simulink model "Crazyflie_NoLinealModel_EB"  (R2020b)
settings: Solver=FixedStepAuto  StartTime=0.0  StopTime=30  FixedStep=0.001  RelTol=1e-3
values from neighbouring files (symbols this model uses):
  fm = 0.2685    [Crazyflie_Model.m]
  we = sqrt((m*g)/(4*CT))    [Crazyflie_Model.m]
undefined symbols (not defined in the file or in its folder): DiscIntNeverNeededParam, Dphi_s, Dphi_T, Dpsi_s, Dtheta_s, KIz, magnitude, MCO, Phi_s, Phi_T, phi_theta_limit, quad, Theta_s, U_s, V_s, X_s, X_T, XY_delta, xyv_lim, Y_s, Yaw_delta, Yaw_s, Yaw_T, Z_delta, Z_s, Z_T
libraries: simulink x16, pid_lib x11
(part 1 of 2)
settings Model: Creator=Rafael  LastModifiedBy=FranciscoJose
settings DataIOCC: LimitDataPoints=on  SaveFormat=Array  SignalLoggingSaveFormat=ModelDataLogs  ReturnWorkspaceOutputs=off
settings OptimizationCC: ExpressionDepthLimit=2147483647  LifeSpan=inf
settings DebuggingCC: UnderspecifiedInitializationDetection=Classic  MergeDetectMultiDrivingBlocksExec=none  SolverPrmCheckMsg=warning  FcnCallInpInsideContextMsg=warning  AllowSymbolicDim=off  StateNameClashWarn=warning  SFUnexpectedBacktrackingDiag=warning  SFNoUnconditionalDefaultTransitionDiag=warning  SFExecutionAtInitializationDiag=none  ArithmeticOperatorsInVariantConditions=warning
settings HardwareCC: ProdBitPerPointer=32  ProdBitPerSizeT=32  ProdBitPerPtrDiffT=32  ProdLargestAtomicFloat=None  ProdIntDivRoundTo=Undefined  ProdEndianess=Unspecified  ProdWordSize=32  ProdHWDeviceType=32-bit Generic
settings ModelReferenceCC: PropagateSignalLabelsOutOfModel=off
settings SFSimCC: SimUseLocalCustomCode=off  CustomCodeUndefinedFunction=UseInterfaceOnly
settings RTWCC: RTWUseLocalCustomCode=off
settings CodeAppCC: StateflowObjectComments=on
settings GRTTargetCC: TargetLangStandard=C89/C90 (ANSI)
settings ConfigComp: CovMetricSettings=dw  CovSaveCumulativeToWorkspaceVar=on  CovSaveSingleToWorkspaceVar=on  CovExternalEMLEnable=off
settings SimscapeCC: SimscapeNormalizeSystem=off
settings ConfigurationSet: Description=SimMechanics 2G

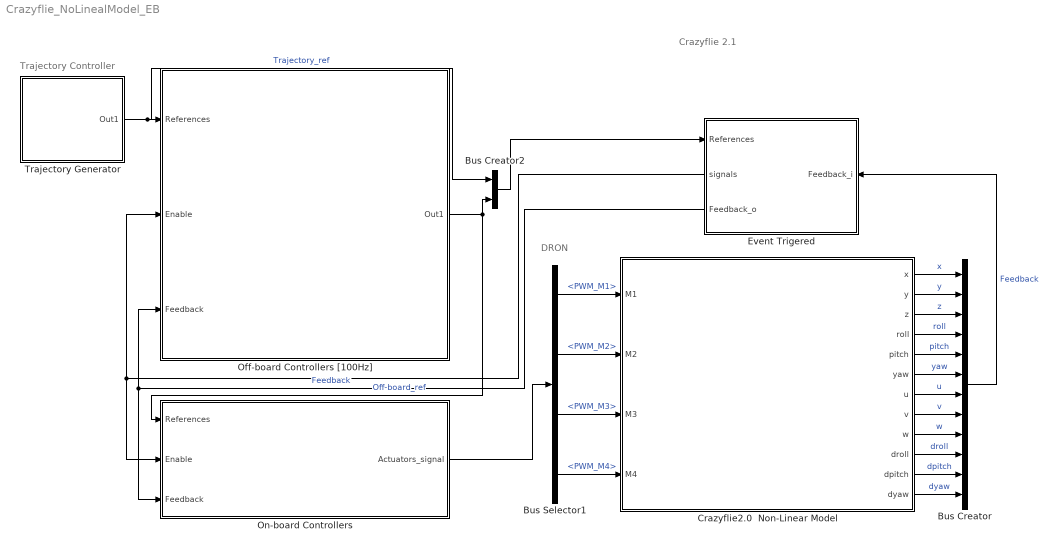
== system Crazyflie_NoLinealModel_EB ==
  note: DRON
  note: Trajectory Controller
  note: Crazyflie 2.1
  Bus Creator : BusCreator  Inputs=12
  Bus Creator2 : BusCreator  Inputs=2
  Bus Selector1 : BusSelector  OutputSignals=PWM_M1,PWM_M2,PWM_M3,PWM_M4
  Crazyflie2.0  Non-Linear Model : Subsystem
      mask Display: image('$imagefile'); % Use "Edit Image" on toolstrip to change.
  Event Trigered : Subsystem
      settings: PortSchema="{\"entries\":[{\"content\":{\"sides\":[{\"content\":{\"connectorIds\":[\"In1\",\"Out1\",\"Out2\"]},\"type\":\"ConnectorPlacement.EquallySpacedRectSide\",\"uuid\":\"5ef058f8-e335-44ad-8d03-d23aa6bafaea\"},{\"content\":{\"connectorIds\":[\"In2\"],\"side\":\"RIGHT\"},\"type\":\"ConnectorPlacement.EquallySpacedRectSide\",\"uuid\":\"829d21a1-bc41-4ced-ab22-24584c4435de\"},{\"content\":{\"connectorIds\":[],\"side\":\"TOP\"},\"type\":\"ConnectorPlacement.EquallySpacedRectSide\",\"uuid\":\"72379b45-c383-4ef8-bce9-8d80bc7025bf\"},{\"content\":{\"connectorIds\":[],\"side\":\"HIDDEN\"},\"type\":\"ConnectorPlacement.EquallySpacedRectSide\",\"uuid\":\"f776fbe7-ec28-4c8f-acaa-997e45e4d7f5\"}]},\"type\":\"ConnectorPlacement.EquallySpacedConnector\",\"uuid\":\"d6c0820c-12f4-49d2-aae7-90f0c967141d\"}],\"packageUris\":[\"http://schema.mathworks.com/mf0/Connector/R2020b\"],\"version\":\"1.0\"}"
  Off-board Controllers [100Hz] : Subsystem
  On-board Controllers : Subsystem
  Trajectory Generator : Subsystem
  wires:
  Crazyflie2.0  Non-Linear Model/11(dpitch) -> Bus Creator/11  "dpitch"
  Crazyflie2.0  Non-Linear Model/3(z) -> Bus Creator/3  "z"
  Crazyflie2.0  Non-Linear Model/12(dyaw) -> Bus Creator/12  "dyaw"
  Crazyflie2.0  Non-Linear Model/4(roll) -> Bus Creator/4  "roll"
  Crazyflie2.0  Non-Linear Model/5(pitch) -> Bus Creator/5  "pitch"
  Crazyflie2.0  Non-Linear Model/6(yaw) -> Bus Creator/6  "yaw"
  Crazyflie2.0  Non-Linear Model/1(x) -> Bus Creator/1  "x"
  Crazyflie2.0  Non-Linear Model/2(y) -> Bus Creator/2  "y"
  Crazyflie2.0  Non-Linear Model/7(u) -> Bus Creator/7  "u"
  Crazyflie2.0  Non-Linear Model/8(v) -> Bus Creator/8  "v"
  Crazyflie2.0  Non-Linear Model/9(w) -> Bus Creator/9  "w"
  Crazyflie2.0  Non-Linear Model/10(droll) -> Bus Creator/10  "droll"
  Event Trigered/2(Feedback_o) -> Off-board Controllers [100Hz]/3(Feedback), On-board Controllers/3(Feedback)  "Feedback"
  Bus Selector1/1 -> Crazyflie2.0  Non-Linear Model/1(M1)  "<PWM_M1>"
  Bus Selector1/2 -> Crazyflie2.0  Non-Linear Model/2(M2)  "<PWM_M2>"
  Bus Selector1/3 -> Crazyflie2.0  Non-Linear Model/3(M3)  "<PWM_M3>"
  Bus Selector1/4 -> Crazyflie2.0  Non-Linear Model/4(M4)  "<PWM_M4>"
  Trajectory Generator/1(Out1) -> Bus Creator2/1, Off-board Controllers [100Hz]/1(References)  "Trajectory_ref"
  Bus Creator2/1 -> Event Trigered/1(References)
  Bus Creator/1 -> Event Trigered/2(Feedback_i)  "Feedback"
  Event Trigered/1(signals) -> On-board Controllers/2(Enable), Off-board Controllers [100Hz]/2(Enable)
  On-board Controllers/1(Actuators_signal) -> Bus Selector1/1
  Off-board Controllers [100Hz]/1(Out1) -> On-board Controllers/1(References), Bus Creator2/2  "Off-board_ref"

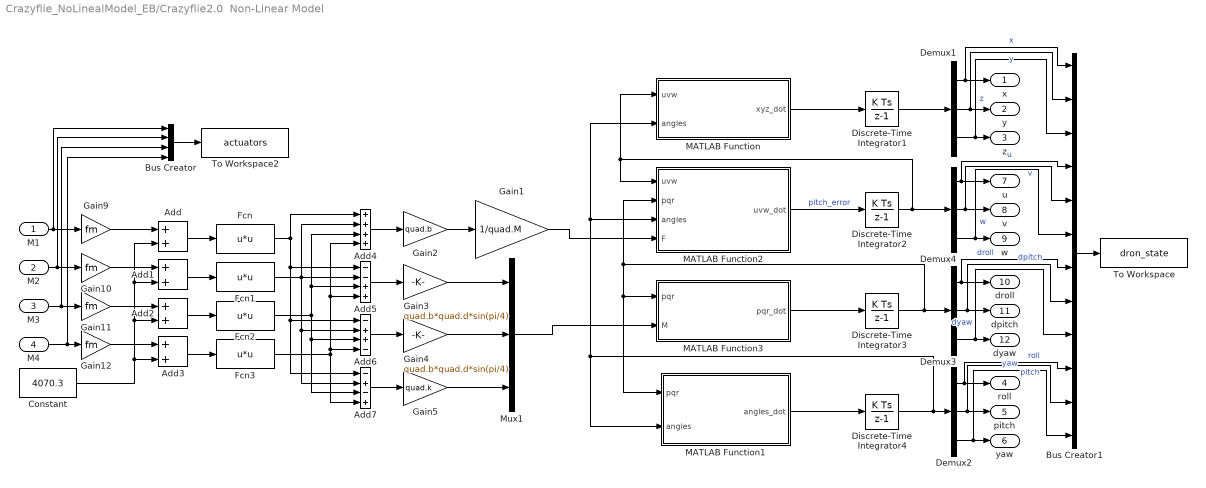
== system Crazyflie_NoLinealModel_EB/Crazyflie2.0  Non-Linear Model ==
  M1 : Inport
  M2 : Inport  Port=2
  M3 : Inport  Port=3
  M4 : Inport  Port=4
  Add{,1..3} (4 alike) : Sum
  Add4 : Sum  Inputs=++++
  Add5 : Sum  Inputs=--++
  Add6 : Sum  Inputs=-++-
  Add7 : Sum  Inputs=-+-+
  Bus Creator : BusCreator  Inputs=4
  Bus Creator1 : BusCreator  Inputs=12
  Constant : Constant  Value=4070.3
  Demux{1..4} (4 alike) : Demux  Outputs=3
  Discrete-Time Integrator{1..4} (4 alike) : DiscreteIntegrator  SampleTime=0.001  ICPrevOutput=DiscIntNeverNeededParam  ICPrevScaledInput=DiscIntNeverNeededParam
  Fcn{,1..3} (4 alike) : Fcn  Expr=u*u
  Gain1 : Gain  Gain=1/quad.M
  Gain{9..12} (4 alike) : Gain  Gain=fm
  Gain2 : Gain  Gain=quad.b
  Gain3 : Gain  Gain=quad.b*quad.d*sin(pi/4)
  Gain4 : Gain  Gain=quad.b*quad.d*sin(pi/4)
  Gain5 : Gain  Gain=quad.k
  MATLAB Function : MATLAB Function  TreatAsAtomicUnit=on
  MATLAB Function1 : MATLAB Function  TreatAsAtomicUnit=on
  MATLAB Function2 : MATLAB Function  TreatAsAtomicUnit=on
  MATLAB Function3 : MATLAB Function  TreatAsAtomicUnit=on
  Mux1 : Mux  Inputs=3
  To Workspace : ToWorkspace  VariableName=dron_state  SaveFormat=Timeseries  SampleTime=-1
  To Workspace2 : ToWorkspace  VariableName=actuators  SaveFormat=Timeseries  SampleTime=-1
  x : Outport
  y : Outport  Port=2
  z : Outport  Port=3
  roll : Outport  Port=4
  pitch : Outport  Port=5
  yaw : Outport  Port=6
  u : Outport  Port=7
  v : Outport  Port=8
  w : Outport  Port=9
  droll : Outport  Port=10
  dpitch : Outport  Port=11
  dyaw : Outport  Port=12
  wires:
  Demux1/1 -> Bus Creator1/1, x/1  "x"
  Demux1/2 -> Bus Creator1/2, y/1  "y"
  Demux1/3 -> Bus Creator1/3, z/1  "z"
  Demux2/1 -> Bus Creator1/10, roll/1  "roll"
  Demux2/2 -> Bus Creator1/11, pitch/1  "pitch"
  Demux2/3 -> Bus Creator1/12, yaw/1  "yaw"
  Demux4/1 -> Bus Creator1/4, u/1  "u"
  Demux4/2 -> Bus Creator1/5, v/1  "v"
  Demux4/3 -> Bus Creator1/6, w/1  "w"
  Demux3/1 -> Bus Creator1/7, droll/1  "droll"
  Demux3/2 -> Bus Creator1/8, dpitch/1  "dpitch"
  Demux3/3 -> Bus Creator1/9, dyaw/1  "dyaw"
  M1/1 -> Bus Creator/1, Gain9/1
  M2/1 -> Gain10/1, Bus Creator/2
  M3/1 -> Bus Creator/3, Gain11/1
  M4/1 -> Bus Creator/4, Gain12/1
  Add/1 -> Fcn/1
  Add1/1 -> Fcn1/1
  Add2/1 -> Fcn2/1
  Add3/1 -> Fcn3/1
  Gain9/1 -> Add/1
  Gain10/1 -> Add1/1
  Gain11/1 -> Add2/1
  Gain12/1 -> Add3/1
  Constant/1 -> Add3/2, Add/2, Add1/2, Add2/2
  Discrete-Time Integrator3/1 -> Demux3/1, MATLAB Function2/2(pqr), MATLAB Function1/1(pqr), MATLAB Function3/1(pqr)
  Discrete-Time Integrator2/1 -> MATLAB Function2/1(uvw), MATLAB Function/1(uvw), Demux4/1
  MATLAB Function3/1(pqr_dot) -> Discrete-Time Integrator3/1
  MATLAB Function1/1(angles_dot) -> Discrete-Time Integrator4/1
  Mux1/1 -> MATLAB Function3/2(M)
  Discrete-Time Integrator4/1 -> Demux2/1, MATLAB Function1/2(angles), MATLAB Function/2(angles), MATLAB Function2/3(angles)
  Discrete-Time Integrator1/1 -> Demux1/1
  MATLAB Function/1(xyz_dot) -> Discrete-Time Integrator1/1
  Gain4/1 -> Mux1/2
  Add6/1 -> Gain4/1
  Gain5/1 -> Mux1/3
  Gain3/1 -> Mux1/1
  Gain1/1 -> MATLAB Function2/4(F)
  Fcn2/1 -> Add4/3, Add5/3, Add7/3, Add6/3
  Add7/1 -> Gain5/1
  Fcn/1 -> Add4/1, Add7/1, Add6/1, Add5/1
  Add5/1 -> Gain3/1
  Fcn3/1 -> Add4/4, Add5/4, Add6/4, Add7/4
  Fcn1/1 -> Add4/2, Add7/2, Add6/2, Add5/2
  Gain2/1 -> Gain1/1
  Add4/1 -> Gain2/1
  MATLAB Function2/1(uvw_dot) -> Discrete-Time Integrator2/1  "pitch_error"
  Bus Creator/1 -> To Workspace2/1
  Bus Creator1/1 -> To Workspace/1

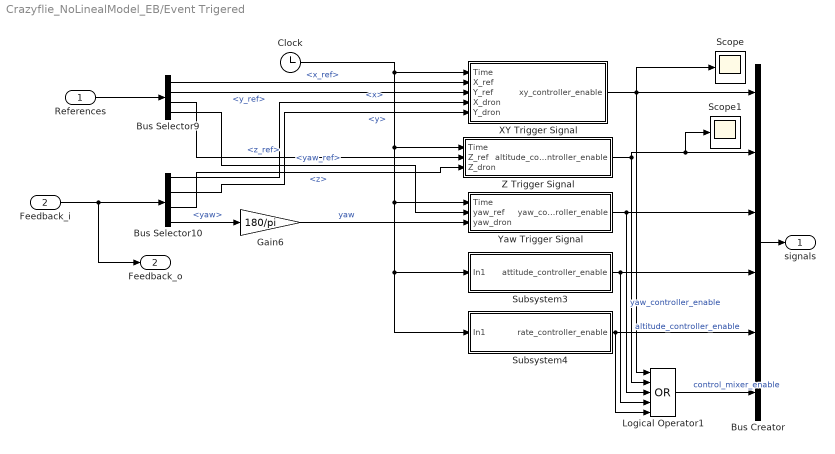
== system Crazyflie_NoLinealModel_EB/Event Trigered ==
  References : Inport
  Feedback_i : Inport  Port=2
  Bus Creator : BusCreator  Inputs=6
  Bus Selector10 : BusSelector  OutputSignals=x,y,z,yaw
  Bus Selector9 : BusSelector  OutputSignals=Trajectory_ref.x_ref,Trajectory_ref.y_ref,Trajectory_ref.z_ref,Trajectory_ref.yaw_ref
  Clock : Clock
  Gain6 : Gain  Gain=180/pi
  Logical Operator1 : Logic  Operator=OR  Inputs=5  AllPortsSameDT=off  OutDataTypeStr=boolean
  Scope : Scope
  Scope1 : Scope
  Subsystem3 : Subsystem
  Subsystem4 : Subsystem
  XY Trigger Signal : Subsystem
  Yaw Trigger Signal : Subsystem
  Z Trigger Signal : Subsystem
  signals : Outport
  Feedback_o : Outport  Port=2
  wires:
  References/1 -> Bus Selector9/1
  Feedback_i/1 -> Bus Selector10/1, Feedback_o/1
  Bus Selector9/1 -> XY Trigger Signal/2(X_ref)  "<x_ref>"
  Bus Selector9/2 -> XY Trigger Signal/3(Y_ref)  "<y_ref>"
  Bus Selector9/4 -> Yaw Trigger Signal/2(yaw_ref)  "<yaw_ref>"
  Bus Selector10/1 -> XY Trigger Signal/4(X_dron)  "<x>"
  Bus Selector10/2 -> XY Trigger Signal/5(Y_dron)  "<y>"
  Bus Selector10/3 -> Z Trigger Signal/3(Z_dron)  "<z>"
  Bus Selector10/4 -> Gain6/1  "<yaw>"
  Bus Selector9/3 -> Z Trigger Signal/2(Z_ref)  "<z_ref>"
  Bus Creator/1 -> signals/1
  Gain6/1 -> Yaw Trigger Signal/3(yaw_dron)  "yaw"
  Logical Operator1/1 -> Bus Creator/6  "control_mixer_enable"
  Z Trigger Signal/1(altitude_controller_enable) -> Scope1/1, Bus Creator/2, Logical Operator1/2  "altitude_controller_enable"
  XY Trigger Signal/1(xy_controller_enable) -> Scope/1, Logical Operator1/1, Bus Creator/1
  Yaw Trigger Signal/1(yaw_controller_enable) -> Logical Operator1/3, Bus Creator/3  "yaw_controller_enable"
  Subsystem3/1(attitude_controller_enable) -> Logical Operator1/4, Bus Creator/4
  Clock/1 -> Subsystem4/1(In1), Subsystem3/1(In1), Yaw Trigger Signal/1(Time), Z Trigger Signal/1(Time), XY Trigger Signal/1(Time)
  Subsystem4/1(rate_controller_enable) -> Logical Operator1/5, Bus Creator/5

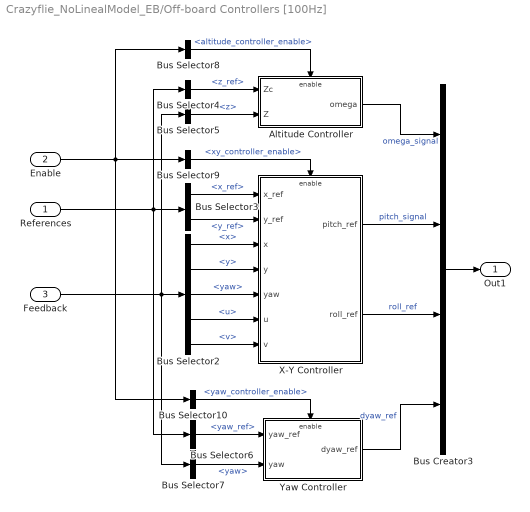
== system Crazyflie_NoLinealModel_EB/Off-board Controllers [100Hz] ==
  References : Inport
  Enable : Inport  Port=2
  Feedback : Inport  Port=3
  Altitude Controller : Subsystem  TreatAsAtomicUnit=on
  Bus Creator3 : BusCreator  Inputs=4
  Bus Selector10 : BusSelector  OutputSignals=yaw_controller_enable
  Bus Selector2 : BusSelector  OutputSignals=x,y,yaw,u,v
  Bus Selector3 : BusSelector  OutputSignals=x_ref,y_ref
  Bus Selector4 : BusSelector  OutputSignals=z_ref
  Bus Selector5 : BusSelector  OutputSignals=z
  Bus Selector6 : BusSelector  OutputSignals=yaw_ref
  Bus Selector7 : BusSelector  OutputSignals=yaw
  Bus Selector8 : BusSelector  OutputSignals=altitude_controller_enable
  Bus Selector9 : BusSelector  OutputSignals=xy_controller_enable
  X-Y Controller : Subsystem  TreatAsAtomicUnit=on
  Yaw Controller : Subsystem  TreatAsAtomicUnit=on
  Out1 : Outport
  wires:
  Bus Selector2/3 -> X-Y Controller/5(yaw)  "<yaw>"
  Bus Selector6/1 -> Yaw Controller/1(yaw_ref)  "<yaw_ref>"
  Bus Selector2/5 -> X-Y Controller/7(v)  "<v>"
  References/1 -> Bus Selector4/1, Bus Selector3/1, Bus Selector6/1
  X-Y Controller/1(pitch_ref) -> Bus Creator3/2  "pitch_signal"
  Enable/1 -> Bus Selector10/1, Bus Selector8/1, Bus Selector9/1
  Feedback/1 -> Bus Selector7/1, Bus Selector5/1, Bus Selector2/1
  Bus Selector2/1 -> X-Y Controller/3(x)  "<x>"
  Bus Selector7/1 -> Yaw Controller/2(yaw)  "<yaw>"
  Bus Selector2/4 -> X-Y Controller/6(u)  "<u>"
  Bus Selector4/1 -> Altitude Controller/1(Zc)  "<z_ref>"
  Bus Selector3/1 -> X-Y Controller/1(x_ref)  "<x_ref>"
  Bus Selector3/2 -> X-Y Controller/2(y_ref)  "<y_ref>"
  Bus Selector2/2 -> X-Y Controller/4(y)  "<y>"
  X-Y Controller/2(roll_ref) -> Bus Creator3/3  "roll_ref"
  Bus Selector5/1 -> Altitude Controller/2(Z)  "<z>"
  Altitude Controller/1(omega) -> Bus Creator3/1  "omega_signal"
  Yaw Controller/1(dyaw_ref) -> Bus Creator3/4  "dyaw_ref"
  Bus Selector9/1 -> X-Y Controller/Enable  "<xy_controller_enable>"
  Bus Selector10/1 -> Yaw Controller/Enable  "<yaw_controller_enable>"
  Bus Selector8/1 -> Altitude Controller/Enable  "<altitude_controller_enable>"
  Bus Creator3/1 -> Out1/1

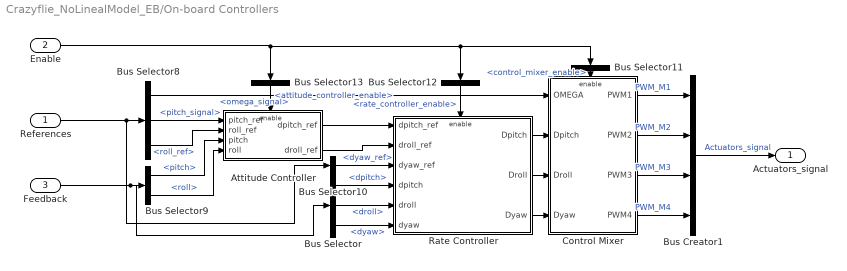
== system Crazyflie_NoLinealModel_EB/On-board Controllers ==
  References : Inport
  Enable : Inport  Port=2
  Feedback : Inport  Port=3
  Attitude Controller : Subsystem  TreatAsAtomicUnit=on
  Bus Creator1 : BusCreator  Inputs=4
  Bus Selector : BusSelector  OutputSignals=dpitch,droll,dyaw
  Bus Selector10 : BusSelector  OutputSignals=dyaw_ref
  Bus Selector11 : BusSelector  OutputSignals=control_mixer_enable
  Bus Selector12 : BusSelector  OutputSignals=rate_controller_enable
  Bus Selector13 : BusSelector  OutputSignals=attitude_controller_enable
  Bus Selector8 : BusSelector  OutputSignals=omega_signal,pitch_signal,roll_ref
  Bus Selector9 : BusSelector  OutputSignals=pitch,roll
  Control Mixer : Subsystem  TreatAsAtomicUnit=on
  Rate Controller : Subsystem  TreatAsAtomicUnit=on
  Actuators_signal : Outport
  wires:
  Bus Creator1/1 -> Actuators_signal/1  "Actuators_signal"
  Bus Selector/2 -> Rate Controller/5(droll)  "<droll>"
  Control Mixer/3(PWM3) -> Bus Creator1/3  "PWM_M3"
  Rate Controller/3(Dyaw) -> Control Mixer/4(Dyaw)
  Enable/1 -> Bus Selector11/1, Bus Selector12/1, Bus Selector13/1
  Bus Selector8/2 -> Attitude Controller/1(pitch_ref)  "<pitch_signal>"
  Bus Selector8/3 -> Attitude Controller/2(roll_ref)  "<roll_ref>"
  References/1 -> Bus Selector8/1, Bus Selector10/1
  Bus Selector12/1 -> Rate Controller/Enable  "<rate_controller_enable>"
  Attitude Controller/2(droll_ref) -> Rate Controller/2(droll_ref)
  Bus Selector10/1 -> Rate Controller/3(dyaw_ref)  "<dyaw_ref>"
  Bus Selector/1 -> Rate Controller/4(dpitch)  "<dpitch>"
  Bus Selector/3 -> Rate Controller/6(dyaw)  "<dyaw>"
  Feedback/1 -> Bus Selector/1, Bus Selector9/1
  Control Mixer/4(PWM4) -> Bus Creator1/4  "PWM_M4"
  Attitude Controller/1(dpitch_ref) -> Rate Controller/1(dpitch_ref)
  Rate Controller/1(Dpitch) -> Control Mixer/2(Dpitch)
  Rate Controller/2(Droll) -> Control Mixer/3(Droll)
  Bus Selector8/1 -> Control Mixer/1(OMEGA)  "<omega_signal>"
  Control Mixer/2(PWM2) -> Bus Creator1/2  "PWM_M2"
  Control Mixer/1(PWM1) -> Bus Creator1/1  "PWM_M1"
  Bus Selector9/2 -> Attitude Controller/4(roll)  "<roll>"
  Bus Selector9/1 -> Attitude Controller/3(pitch)  "<pitch>"
  Bus Selector11/1 -> Control Mixer/Enable  "<control_mixer_enable>"
  Bus Selector13/1 -> Attitude Controller/Enable  "<attitude_controller_enable>"

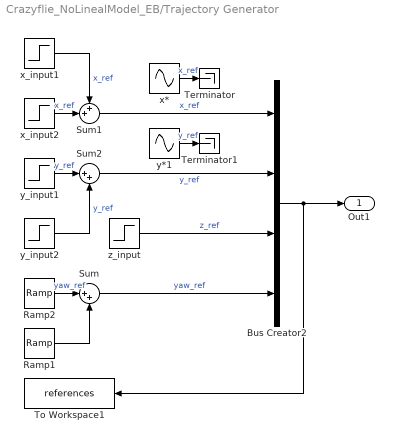
== system Crazyflie_NoLinealModel_EB/Trajectory Generator ==
  Bus Creator2 : BusCreator  Inputs=4
  Ramp1 : simulink/Sources/Ramp  slope=-pi/3  start=10  InitialOutput=0
  Ramp2 : simulink/Sources/Ramp  slope=pi/3  start=0  InitialOutput=0
  Sum : Sum  Inputs=|++
  Sum1 : Sum  Inputs=++|
  Sum2 : Sum  Inputs=|++
  Terminator : Terminator
  Terminator1 : Terminator
  To Workspace1 : ToWorkspace  VariableName=references  SaveFormat=Timeseries  SampleTime=-1
  x* : Sin  Amplitude=0.8  Frequency=2*pi*0.085  Phase=0-0.1  SampleTime=0
  x_input1 : Step  Time=6  SampleTime=0
  x_input2 : Step  Time=18  After=-1  SampleTime=0
  y*1 : Sin  Amplitude=0.8  Frequency=2*pi*0.085  Phase=pi/2-0.1  SampleTime=0
  y_input1 : Step  Time=12  SampleTime=0
  y_input2 : Step  Time=24  After=-1  SampleTime=0
  z_input : Step  Time=0  SampleTime=0
  Out1 : Outport
  wires:
  z_input/1 -> Bus Creator2/3  "z_ref"
  Sum1/1 -> Bus Creator2/1  "x_ref"
  Ramp1/1 -> Sum/2
  Sum2/1 -> Bus Creator2/2  "y_ref"
  Bus Creator2/1 -> To Workspace1/1, Out1/1
  Sum/1 -> Bus Creator2/4  "yaw_ref"
  Ramp2/1 -> Sum/1  "yaw_ref"
  x_input2/1 -> Sum1/2  "x_ref"
  x_input1/1 -> Sum1/1  "x_ref"
  y_input1/1 -> Sum2/1  "y_ref"
  y_input2/1 -> Sum2/2  "y_ref"
  x*/1 -> Terminator/1  "x_ref"
  y*1/1 -> Terminator1/1  "y_ref"

== system Crazyflie_NoLinealModel_EB/Event Trigered/Subsystem3 ==
  In1 : Inport
  Compare To Constant4 : simulink/Logic and Bit Operations/Compare To Constant  relop=>=  const=Phi_T  OutDataTypeStr=boolean
  If Action Subsystem4 : Subsystem  TreatAsAtomicUnit=on
  Memory4 : Memory
  Sum8 : Sum  Inputs=|+-
  attitude_controller_enable : Outport
  wires:
  In1/1 -> Sum8/1, If Action Subsystem4/1(In2)
  If Action Subsystem4/1(Out2) -> Memory4/1
  Compare To Constant4/1 -> attitude_controller_enable/1, If Action Subsystem4/Enable  "attitude_controller_enable"
  Memory4/1 -> Sum8/2
  Sum8/1 -> Compare To Constant4/1

== system Crazyflie_NoLinealModel_EB/Event Trigered/Subsystem4 ==
  In1 : Inport
  Compare To Constant4 : simulink/Logic and Bit Operations/Compare To Constant  relop=>=  const=Dphi_T  OutDataTypeStr=boolean
  If Action Subsystem4 : Subsystem  TreatAsAtomicUnit=on
  Memory4 : Memory
  Sum8 : Sum  Inputs=|+-
  rate_controller_enable : Outport
  wires:
  In1/1 -> Sum8/1, If Action Subsystem4/1(In2)
  Sum8/1 -> Compare To Constant4/1
  If Action Subsystem4/1(Out2) -> Memory4/1
  Compare To Constant4/1 -> rate_controller_enable/1, If Action Subsystem4/Enable  "rate_controller_enable"
  Memory4/1 -> Sum8/2

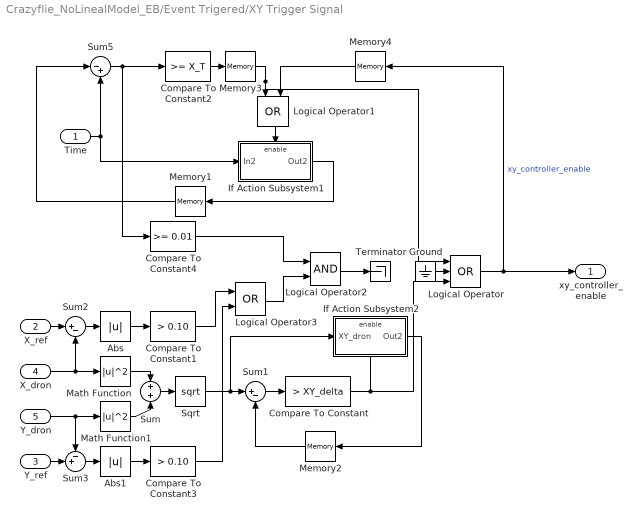
== system Crazyflie_NoLinealModel_EB/Event Trigered/XY Trigger Signal ==
  Time : Inport
  X_ref : Inport  Port=2
  Y_ref : Inport  Port=3
  X_dron : Inport  Port=4
  Y_dron : Inport  Port=5
  Abs : Abs
  Abs1 : Abs
  Compare To Constant : simulink/Logic and Bit Operations/Compare To Constant  relop=>  const=XY_delta  OutDataTypeStr=boolean
  Compare To Constant1 : simulink/Logic and Bit Operations/Compare To Constant  relop=>  const=0.10  OutDataTypeStr=boolean
  Compare To Constant2 : simulink/Logic and Bit Operations/Compare To Constant  relop=>=  const=X_T  OutDataTypeStr=boolean
  Compare To Constant3 : simulink/Logic and Bit Operations/Compare To Constant  relop=>  const=0.10  OutDataTypeStr=boolean
  Compare To Constant4 : simulink/Logic and Bit Operations/Compare To Constant  relop=>=  const=0.01  OutDataTypeStr=boolean
  Ground : Ground
  If Action Subsystem1 : Subsystem  TreatAsAtomicUnit=on
  If Action Subsystem2 : Subsystem  TreatAsAtomicUnit=on
  Logical Operator : Logic  Operator=OR  Inputs=3  AllPortsSameDT=off  OutDataTypeStr=boolean
  Logical Operator1 : Logic  Operator=OR  AllPortsSameDT=off  OutDataTypeStr=boolean
  Logical Operator2 : Logic  AllPortsSameDT=off  OutDataTypeStr=boolean
  Logical Operator3 : Logic  Operator=OR  AllPortsSameDT=off  OutDataTypeStr=boolean
  Math Function : Math  Operator=magnitude^2  SaturateOnIntegerOverflow=on
  Math Function1 : Math  Operator=magnitude^2  SaturateOnIntegerOverflow=on
  Memory{1..4} (4 alike) : Memory
  Sqrt : Sqrt  SaturateOnIntegerOverflow=on
  Sum : Sum
  Sum1 : Sum  Inputs=|+-
  Sum2 : Sum  Inputs=|+-
  Sum3 : Sum  Inputs=-+|
  Sum5 : Sum  Inputs=|-+
  Terminator : Terminator
  xy_controller_enable : Outport
  wires:
  Logical Operator/1 -> Memory4/1, xy_controller_enable/1  "xy_controller_enable"
  Compare To Constant/1 -> Logical Operator/3, If Action Subsystem2/Enable
  Math Function/1 -> Sum/1
  Math Function1/1 -> Sum/2
  Sum/1 -> Sqrt/1
  Sum1/1 -> Compare To Constant/1
  Memory4/1 -> Logical Operator1/2
  Memory3/1 -> Logical Operator/1, Logical Operator1/1
  Logical Operator1/1 -> If Action Subsystem1/Enable
  If Action Subsystem1/1(Out2) -> Memory1/1
  Time/1 -> Sum5/2, If Action Subsystem1/1(In2)
  Sum5/1 -> Compare To Constant4/1, Compare To Constant2/1
  Compare To Constant2/1 -> Memory3/1
  Memory1/1 -> Sum5/1
  X_dron/1 -> Math Function/1, Sum2/2
  Y_dron/1 -> Math Function1/1, Sum3/1
  Sqrt/1 -> If Action Subsystem2/1(XY_dron), Sum1/1
  If Action Subsystem2/1(Out2) -> Memory2/1
  Memory2/1 -> Sum1/2
  Y_ref/1 -> Sum3/2
  X_ref/1 -> Sum2/1
  Sum2/1 -> Abs/1
  Sum3/1 -> Abs1/1
  Compare To Constant1/1 -> Logical Operator3/1
  Abs/1 -> Compare To Constant1/1
  Compare To Constant3/1 -> Logical Operator3/2
  Abs1/1 -> Compare To Constant3/1
  Compare To Constant4/1 -> Logical Operator2/1
  Logical Operator3/1 -> Logical Operator2/2
  Logical Operator2/1 -> Terminator/1
  Ground/1 -> Logical Operator/2

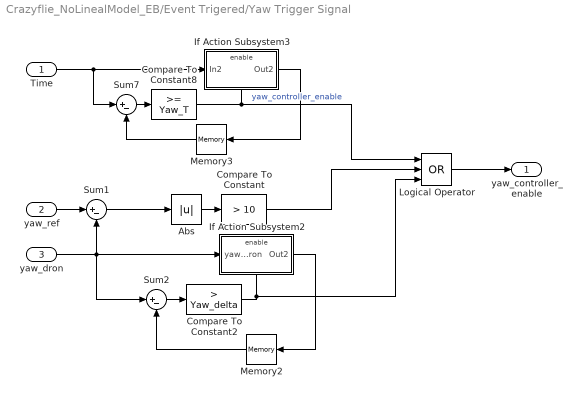
== system Crazyflie_NoLinealModel_EB/Event Trigered/Yaw Trigger Signal ==
  Time : Inport
  yaw_ref : Inport  Port=2
  yaw_dron : Inport  Port=3
  Abs : Abs
  Compare To Constant : simulink/Logic and Bit Operations/Compare To Constant  relop=>  const=10  OutDataTypeStr=boolean
  Compare To Constant2 : simulink/Logic and Bit Operations/Compare To Constant  relop=>  const=Yaw_delta  OutDataTypeStr=boolean
  Compare To Constant8 : simulink/Logic and Bit Operations/Compare To Constant  relop=>=  const=Yaw_T  OutDataTypeStr=boolean
  If Action Subsystem2 : Subsystem  TreatAsAtomicUnit=on
  If Action Subsystem3 : Subsystem  TreatAsAtomicUnit=on
  Logical Operator : Logic  Operator=OR  Inputs=3  AllPortsSameDT=off  OutDataTypeStr=boolean
  Memory2 : Memory
  Memory3 : Memory
  Sum1 : Sum  Inputs=|+-
  Sum2 : Sum  Inputs=|+-
  Sum7 : Sum  Inputs=|+-
  yaw_controller_enable : Outport
  wires:
  Time/1 -> Sum7/1, If Action Subsystem3/1(In2)
  If Action Subsystem3/1(Out2) -> Memory3/1
  Sum7/1 -> Compare To Constant8/1
  Memory3/1 -> Sum7/2
  Compare To Constant/1 -> Logical Operator/2
  Abs/1 -> Compare To Constant/1
  Logical Operator/1 -> yaw_controller_enable/1
  Compare To Constant8/1 -> If Action Subsystem3/Enable, Logical Operator/1  "yaw_controller_enable"
  yaw_ref/1 -> Sum1/1
  Sum1/1 -> Abs/1
  Sum2/1 -> Compare To Constant2/1
  Memory2/1 -> Sum2/2
  Compare To Constant2/1 -> Logical Operator/3, If Action Subsystem2/Enable
  yaw_dron/1 -> Sum2/1, If Action Subsystem2/1(yaw_dron), Sum1/2
  If Action Subsystem2/1(Out2) -> Memory2/1

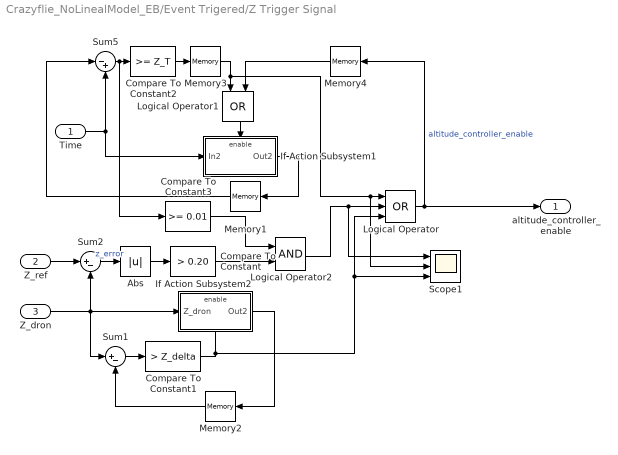
== system Crazyflie_NoLinealModel_EB/Event Trigered/Z Trigger Signal ==
  Time : Inport
  Z_ref : Inport  Port=2
  Z_dron : Inport  Port=3
  Abs : Abs
  Compare To Constant : simulink/Logic and Bit Operations/Compare To Constant  relop=>  const=0.20  OutDataTypeStr=boolean
  Compare To Constant1 : simulink/Logic and Bit Operations/Compare To Constant  relop=>  const=Z_delta  OutDataTypeStr=boolean
  Compare To Constant2 : simulink/Logic and Bit Operations/Compare To Constant  relop=>=  const=Z_T  OutDataTypeStr=boolean
  Compare To Constant3 : simulink/Logic and Bit Operations/Compare To Constant  relop=>=  const=0.01  OutDataTypeStr=boolean
  If Action Subsystem1 : Subsystem  TreatAsAtomicUnit=on
  If Action Subsystem2 : Subsystem  TreatAsAtomicUnit=on
  Logical Operator : Logic  Operator=OR  Inputs=3  AllPortsSameDT=off  OutDataTypeStr=boolean
  Logical Operator1 : Logic  Operator=OR  AllPortsSameDT=off  OutDataTypeStr=boolean
  Logical Operator2 : Logic  AllPortsSameDT=off  OutDataTypeStr=boolean
  Memory{1..4} (4 alike) : Memory
  Scope1 : Scope  NumInputPorts=3
  Sum1 : Sum  Inputs=|+-
  Sum2 : Sum  Inputs=|+-
  Sum5 : Sum  Inputs=|-+
  altitude_controller_enable : Outport
  wires:
  Sum5/1 -> Compare To Constant3/1, Compare To Constant2/1
  Time/1 -> Sum5/2, If Action Subsystem1/1(In2)
  If Action Subsystem1/1(Out2) -> Memory1/1
  Logical Operator/1 -> altitude_controller_enable/1, Memory4/1  "altitude_controller_enable"
  Memory1/1 -> Sum5/1
  Abs/1 -> Compare To Constant/1
  Sum2/1 -> Abs/1  "z_error"
  Logical Operator1/1 -> If Action Subsystem1/Enable
  Z_ref/1 -> Sum2/1
  Z_dron/1 -> Sum2/2, Sum1/1, If Action Subsystem2/1(Z_dron)
  Sum1/1 -> Compare To Constant1/1
  Memory2/1 -> Sum1/2
  If Action Subsystem2/1(Out2) -> Memory2/1
  Compare To Constant1/1 -> Scope1/3, Logical Operator/3, If Action Subsystem2/Enable
  Memory3/1 -> Scope1/2, Logical Operator/1, Logical Operator1/1
  Compare To Constant2/1 -> Memory3/1
  Memory4/1 -> Logical Operator1/2
  Compare To Constant/1 -> Logical Operator2/2
  Logical Operator2/1 -> Scope1/1, Logical Operator/2
  Compare To Constant3/1 -> Logical Operator2/1

== system Crazyflie_NoLinealModel_EB/Off-board Controllers [100Hz]/Altitude Controller ==
  Zc : Inport
  Z : Inport  Port=2
  Enable : EnablePort
  Bus Creator : BusCreator  Inputs=5
  Constant : Constant  Value=we
  Constant1 : Constant  Value=4070.3
  Gain : Gain  Gain=1/fm
  PID Controller : pid_lib/PID Controller  Controller=PID  Form=Parallel  TimeDomain=Continuous-time  UseExternalTs=off  SampleTime=-1  IntegratorMethod=Forward Euler  FilterMethod=Forward Euler  ControllerParametersSource=internal  P=Z_s(1)  I=Z_s(2)  D=Z_s(3)  UseFilter=on  N=100  TunerSelectOption=Transfer Function Based (PID Tuner App)  InitialConditionSource=internal  InitialConditionForIntegrator=0  InitialConditionForFilter=0  DifferentiatorICPrevScaledInput=0  ExternalReset=none  TrackingMode=off  Kt=1  LimitOutput=on  SatLimitsSource=internal  UpperSaturationLimit=15000  LowerSaturationLimit=-20000  LinearizeAsGain=on  AntiWindupMode=none  Kb=1/sqrt(KIz)  POutMin=[]  POutMax=[]  IOutMin=[]  IOutMax=[]  DOutMin=[]  DOutMax=[]  NOutMin=[]  NOutMax=[]  SumOutMin=[]  SumOutMax=[]  SaturationOutMin=[]  SaturationOutMax=[]  PParamMin=[]  PParamMax=[]  IParamMin=[]  IParamMax=[]  DParamMin=[]  DParamMax=[]  NParamMin=[]  NParamMax=[]  KbParamMin=[]  KbParamMax=[]  KtParamMin=[]  KtParamMax=[]  KbOutMin=[]  KbOutMax=[]  KtOutMin=[]  KtOutMax=[]  IntegratorOutMin=[]  IntegratorOutMax=[]  FilterOutMin=[]  FilterOutMax=[]  SumI1OutMin=[]  SumI1OutMax=[]  SumI2OutMin=[]  SumI2OutMax=[]  SumI3OutMin=[]  SumI3OutMax=[]  SumI4OutMin=[]  SumI4OutMax=[]  SumDOutMin=[]  SumDOutMax=[]  DifferentiatorOutMin=[]  DifferentiatorOutMax=[]  FilterDiffOutCoefMin=[]  FilterDiffOutCoefMax=[]  ReciprocalOutMin=[]  ReciprocalOutMax=[]  SumDenOutMin=[]  SumDenOutMax=[]  SumNumOutMin=[]  SumNumOutMax=[]  DivideOutMin=[]  DivideOutMax=[]  UdiffTsProdOutMin=[]  UdiffTsProdOutMax=[]  NTsProdOutMin=[]  NTsProdOutMax=[]  UintegralTsProdOutMin=[]  UintegralTsProdOutMax=[]  UngainTsProdOutMin=[]  UngainTsProdOutMax=[]  IntegratorContinuousStateAttributes=''  IntegratorStateMustResolveToSignalObject=off  IntegratorRTWStateStorageClass=Auto  FilterContinuousStateAttributes=''  FilterStateMustResolveToSignalObject=off  FilterRTWStateStorageClass=Auto  ParallelPVariant=InternalParameters  IdealPVariant=Disabled  IVariant=InternalParameters  DVariant=InternalParameters  IntegratorVariant=Continuous  SatVariant=Enabled  AWVariant=Passthrough  PCopyVariant=Disabled  TRVariant=Disabled  FdbkBlocksVariant=Forward  IdealPFdbkVariant=Disabled  SatFdbkVariant=Disabled  DerivativeFilterVariant=ContFilter  NVariant=InternalParameters  NCopyVariant=Disabled  FilterICVariant=InternalICsFilter  IntegratorICVariant=InternalICs  ExternalResetVariant=Disabled  TRSumVariant=Passthrough  SumFdbkVariant=Disabled  SumVariant=Sum_PID  TsampFilterVariant=InternalTs  TsampNgainVariant=Passthrough  TsampIntegralVariant=Passthrough  ExternalSaturationOutDataTypeStr=Inherit: Same as second input
  Sum : Sum  Inputs=|++
  Sum1 : Sum  Inputs=|+-
  Sum2 : Sum  Inputs=|+-
  To Workspace : ToWorkspace  VariableName=altitude_controller  SaveFormat=Timeseries  SampleTime=-1
  omega : Outport
  wires:
  Zc/1 -> Bus Creator/1, Sum1/1
  Bus Creator/1 -> To Workspace/1
  Z/1 -> Bus Creator/2, Sum1/2
  Gain/1 -> Sum/2
  PID Controller/1 -> Bus Creator/4, Sum/1  "delta_omega"
  Constant1/1 -> Sum2/2
  Sum2/1 -> Gain/1
  Sum1/1 -> PID Controller/1, Bus Creator/3  "z_error"
  Sum/1 -> Bus Creator/5, omega/1  "omega"
  Constant/1 -> Sum2/1

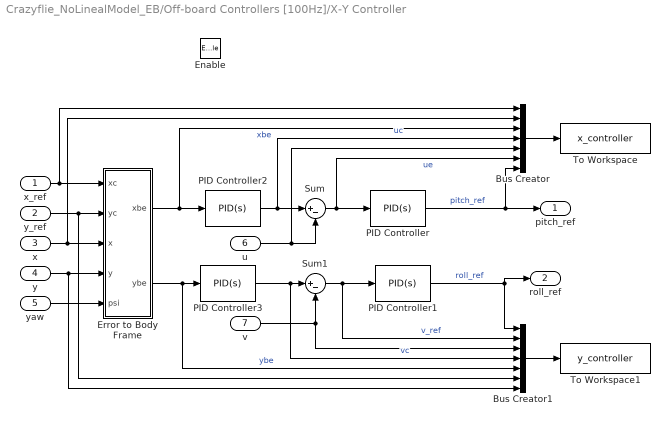
== system Crazyflie_NoLinealModel_EB/Off-board Controllers [100Hz]/X-Y Controller ==
  x_ref : Inport
  y_ref : Inport  Port=2
  x : Inport  Port=3
  y : Inport  Port=4
  yaw : Inport  Port=5
  u : Inport  Port=6
  v : Inport  Port=7
  Enable : EnablePort
  Bus Creator : BusCreator  Inputs=7
  Bus Creator1 : BusCreator  Inputs=7
  Error to Body Frame : MATLAB Function  TreatAsAtomicUnit=on
  PID Controller : pid_lib/PID Controller  Controller=PID  Form=Parallel  TimeDomain=Continuous-time  UseExternalTs=off  SampleTime=-1  IntegratorMethod=Forward Euler  FilterMethod=Forward Euler  ControllerParametersSource=internal  P=U_s(1)  I=U_s(2)  D=U_s(3)  UseFilter=on  N=100  TunerSelectOption=Transfer Function Based (PID Tuner App)  InitialConditionSource=internal  InitialConditionForIntegrator=0  InitialConditionForFilter=0  DifferentiatorICPrevScaledInput=0  ExternalReset=none  TrackingMode=off  Kt=1  LimitOutput=on  SatLimitsSource=internal  UpperSaturationLimit=xyv_lim  LowerSaturationLimit=-xyv_lim  LinearizeAsGain=on  AntiWindupMode=back-calculation  Kb=1/sqrt(U_s(2))  POutMin=[]  POutMax=[]  IOutMin=[]  IOutMax=[]  DOutMin=[]  DOutMax=[]  NOutMin=[]  NOutMax=[]  SumOutMin=[]  SumOutMax=[]  SaturationOutMin=[]  SaturationOutMax=[]  PParamMin=[]  PParamMax=[]  IParamMin=[]  IParamMax=[]  DParamMin=[]  DParamMax=[]  NParamMin=[]  NParamMax=[]  KbParamMin=[]  KbParamMax=[]  KtParamMin=[]  KtParamMax=[]  KbOutMin=[]  KbOutMax=[]  KtOutMin=[]  KtOutMax=[]  IntegratorOutMin=[]  IntegratorOutMax=[]  FilterOutMin=[]  FilterOutMax=[]  SumI1OutMin=[]  SumI1OutMax=[]  SumI2OutMin=[]  SumI2OutMax=[]  SumI3OutMin=[]  SumI3OutMax=[]  SumI4OutMin=[]  SumI4OutMax=[]  SumDOutMin=[]  SumDOutMax=[]  DifferentiatorOutMin=[]  DifferentiatorOutMax=[]  FilterDiffOutCoefMin=[]  FilterDiffOutCoefMax=[]  ReciprocalOutMin=[]  ReciprocalOutMax=[]  SumDenOutMin=[]  SumDenOutMax=[]  SumNumOutMin=[]  SumNumOutMax=[]  DivideOutMin=[]  DivideOutMax=[]  UdiffTsProdOutMin=[]  UdiffTsProdOutMax=[]  NTsProdOutMin=[]  NTsProdOutMax=[]  UintegralTsProdOutMin=[]  UintegralTsProdOutMax=[]  UngainTsProdOutMin=[]  UngainTsProdOutMax=[]  IntegratorContinuousStateAttributes=''  IntegratorStateMustResolveToSignalObject=off  IntegratorRTWStateStorageClass=Auto  FilterContinuousStateAttributes=''  FilterStateMustResolveToSignalObject=off  FilterRTWStateStorageClass=Auto  ParallelPVariant=InternalParameters  IdealPVariant=Disabled  IVariant=InternalParameters  DVariant=InternalParameters  IntegratorVariant=Continuous  SatVariant=Enabled  AWVariant=BackCalculation  PCopyVariant=Disabled  TRVariant=Disabled  FdbkBlocksVariant=Forward  IdealPFdbkVariant=Disabled  SatFdbkVariant=Disabled  DerivativeFilterVariant=ContFilter  NVariant=InternalParameters  NCopyVariant=Disabled  FilterICVariant=InternalICsFilter  IntegratorICVariant=InternalICs  ExternalResetVariant=Disabled  TRSumVariant=Passthrough  SumFdbkVariant=Disabled  SumVariant=Sum_PID  TsampFilterVariant=InternalTs  TsampNgainVariant=Passthrough  TsampIntegralVariant=Passthrough  ExternalSaturationOutDataTypeStr=Inherit: Same as second input
  PID Controller1 : pid_lib/PID Controller  Controller=PID  Form=Parallel  TimeDomain=Continuous-time  UseExternalTs=off  SampleTime=-1  IntegratorMethod=Forward Euler  FilterMethod=Forward Euler  ControllerParametersSource=internal  P=V_s(1)  I=V_s(2)  D=V_s(3)  UseFilter=on  N=100  TunerSelectOption=Transfer Function Based (PID Tuner App)  InitialConditionSource=internal  InitialConditionForIntegrator=0  InitialConditionForFilter=0  DifferentiatorICPrevScaledInput=0  ExternalReset=none  TrackingMode=off  Kt=1  LimitOutput=on  SatLimitsSource=internal  UpperSaturationLimit=xyv_lim  LowerSaturationLimit=-xyv_lim  LinearizeAsGain=on  AntiWindupMode=back-calculation  Kb=1/sqrt(abs(V_s(2)))  POutMin=[]  POutMax=[]  IOutMin=[]  IOutMax=[]  DOutMin=[]  DOutMax=[]  NOutMin=[]  NOutMax=[]  SumOutMin=[]  SumOutMax=[]  SaturationOutMin=[]  SaturationOutMax=[]  PParamMin=[]  PParamMax=[]  IParamMin=[]  IParamMax=[]  DParamMin=[]  DParamMax=[]  NParamMin=[]  NParamMax=[]  KbParamMin=[]  KbParamMax=[]  KtParamMin=[]  KtParamMax=[]  KbOutMin=[]  KbOutMax=[]  KtOutMin=[]  KtOutMax=[]  IntegratorOutMin=[]  IntegratorOutMax=[]  FilterOutMin=[]  FilterOutMax=[]  SumI1OutMin=[]  SumI1OutMax=[]  SumI2OutMin=[]  SumI2OutMax=[]  SumI3OutMin=[]  SumI3OutMax=[]  SumI4OutMin=[]  SumI4OutMax=[]  SumDOutMin=[]  SumDOutMax=[]  DifferentiatorOutMin=[]  DifferentiatorOutMax=[]  FilterDiffOutCoefMin=[]  FilterDiffOutCoefMax=[]  ReciprocalOutMin=[]  ReciprocalOutMax=[]  SumDenOutMin=[]  SumDenOutMax=[]  SumNumOutMin=[]  SumNumOutMax=[]  DivideOutMin=[]  DivideOutMax=[]  UdiffTsProdOutMin=[]  UdiffTsProdOutMax=[]  NTsProdOutMin=[]  NTsProdOutMax=[]  UintegralTsProdOutMin=[]  UintegralTsProdOutMax=[]  UngainTsProdOutMin=[]  UngainTsProdOutMax=[]  IntegratorContinuousStateAttributes=''  IntegratorStateMustResolveToSignalObject=off  IntegratorRTWStateStorageClass=Auto  FilterContinuousStateAttributes=''  FilterStateMustResolveToSignalObject=off  FilterRTWStateStorageClass=Auto  ParallelPVariant=InternalParameters  IdealPVariant=Disabled  IVariant=InternalParameters  DVariant=InternalParameters  IntegratorVariant=Continuous  SatVariant=Enabled  AWVariant=BackCalculation  PCopyVariant=Disabled  TRVariant=Disabled  FdbkBlocksVariant=Forward  IdealPFdbkVariant=Disabled  SatFdbkVariant=Disabled  DerivativeFilterVariant=ContFilter  NVariant=InternalParameters  NCopyVariant=Disabled  FilterICVariant=InternalICsFilter  IntegratorICVariant=InternalICs  ExternalResetVariant=Disabled  TRSumVariant=Passthrough  SumFdbkVariant=Disabled  SumVariant=Sum_PID  TsampFilterVariant=InternalTs  TsampNgainVariant=Passthrough  TsampIntegralVariant=Passthrough  ExternalSaturationOutDataTypeStr=Inherit: Same as second input
  PID Controller2 : pid_lib/PID Controller  Controller=PID  Form=Parallel  TimeDomain=Continuous-time  UseExternalTs=off  SampleTime=-1  IntegratorMethod=Forward Euler  FilterMethod=Forward Euler  ControllerParametersSource=internal  P=X_s(1)  I=X_s(2)  D=X_s(3)  UseFilter=on  N=100  TunerSelectOption=Transfer Function Based (PID Tuner App)  InitialConditionSource=internal  InitialConditionForIntegrator=0  InitialConditionForFilter=0  DifferentiatorICPrevScaledInput=0  ExternalReset=none  TrackingMode=off  Kt=1  LimitOutput=off  SatLimitsSource=internal  UpperSaturationLimit=1.5  LowerSaturationLimit=-1.5  LinearizeAsGain=on  AntiWindupMode=none  Kb=1/sqrt(2)  POutMin=[]  POutMax=[]  IOutMin=[]  IOutMax=[]  DOutMin=[]  DOutMax=[]  NOutMin=[]  NOutMax=[]  SumOutMin=[]  SumOutMax=[]  SaturationOutMin=[]  SaturationOutMax=[]  PParamMin=[]  PParamMax=[]  IParamMin=[]  IParamMax=[]  DParamMin=[]  DParamMax=[]  NParamMin=[]  NParamMax=[]  KbParamMin=[]  KbParamMax=[]  KtParamMin=[]  KtParamMax=[]  KbOutMin=[]  KbOutMax=[]  KtOutMin=[]  KtOutMax=[]  IntegratorOutMin=[]  IntegratorOutMax=[]  FilterOutMin=[]  FilterOutMax=[]  SumI1OutMin=[]  SumI1OutMax=[]  SumI2OutMin=[]  SumI2OutMax=[]  SumI3OutMin=[]  SumI3OutMax=[]  SumI4OutMin=[]  SumI4OutMax=[]  SumDOutMin=[]  SumDOutMax=[]  DifferentiatorOutMin=[]  DifferentiatorOutMax=[]  FilterDiffOutCoefMin=[]  FilterDiffOutCoefMax=[]  ReciprocalOutMin=[]  ReciprocalOutMax=[]  SumDenOutMin=[]  SumDenOutMax=[]  SumNumOutMin=[]  SumNumOutMax=[]  DivideOutMin=[]  DivideOutMax=[]  UdiffTsProdOutMin=[]  UdiffTsProdOutMax=[]  NTsProdOutMin=[]  NTsProdOutMax=[]  UintegralTsProdOutMin=[]  UintegralTsProdOutMax=[]  UngainTsProdOutMin=[]  UngainTsProdOutMax=[]  IntegratorContinuousStateAttributes=''  IntegratorStateMustResolveToSignalObject=off  IntegratorRTWStateStorageClass=Auto  FilterContinuousStateAttributes=''  FilterStateMustResolveToSignalObject=off  FilterRTWStateStorageClass=Auto  ParallelPVariant=InternalParameters  IdealPVariant=Disabled  IVariant=InternalParameters  DVariant=InternalParameters  IntegratorVariant=Continuous  SatVariant=Disabled  AWVariant=Passthrough  PCopyVariant=Disabled  TRVariant=Disabled  FdbkBlocksVariant=Forward  IdealPFdbkVariant=Disabled  SatFdbkVariant=Disabled  DerivativeFilterVariant=ContFilter  NVariant=InternalParameters  NCopyVariant=Disabled  FilterICVariant=InternalICsFilter  IntegratorICVariant=InternalICs  ExternalResetVariant=Disabled  TRSumVariant=Passthrough  SumFdbkVariant=Disabled  SumVariant=Sum_PID  TsampFilterVariant=InternalTs  TsampNgainVariant=Passthrough  TsampIntegralVariant=Passthrough  ExternalSaturationOutDataTypeStr=Inherit: Same as second input
  PID Controller3 : pid_lib/PID Controller  Controller=PID  Form=Parallel  TimeDomain=Continuous-time  UseExternalTs=off  SampleTime=-1  IntegratorMethod=Forward Euler  FilterMethod=Forward Euler  ControllerParametersSource=internal  P=Y_s(1)  I=Y_s(2)  D=Y_s(3)  UseFilter=on  N=100  TunerSelectOption=Transfer Function Based (PID Tuner App)  InitialConditionSource=internal  InitialConditionForIntegrator=0  InitialConditionForFilter=0  DifferentiatorICPrevScaledInput=0  ExternalReset=none  TrackingMode=off  Kt=1  LimitOutput=off  SatLimitsSource=internal  UpperSaturationLimit=1.5  LowerSaturationLimit=-1.5  LinearizeAsGain=on  AntiWindupMode=none  Kb=1/sqrt(2)  POutMin=[]  POutMax=[]  IOutMin=[]  IOutMax=[]  DOutMin=[]  DOutMax=[]  NOutMin=[]  NOutMax=[]  SumOutMin=[]  SumOutMax=[]  SaturationOutMin=[]  SaturationOutMax=[]  PParamMin=[]  PParamMax=[]  IParamMin=[]  IParamMax=[]  DParamMin=[]  DParamMax=[]  NParamMin=[]  NParamMax=[]  KbParamMin=[]  KbParamMax=[]  KtParamMin=[]  KtParamMax=[]  KbOutMin=[]  KbOutMax=[]  KtOutMin=[]  KtOutMax=[]  IntegratorOutMin=[]  IntegratorOutMax=[]  FilterOutMin=[]  FilterOutMax=[]  SumI1OutMin=[]  SumI1OutMax=[]  SumI2OutMin=[]  SumI2OutMax=[]  SumI3OutMin=[]  SumI3OutMax=[]  SumI4OutMin=[]  SumI4OutMax=[]  SumDOutMin=[]  SumDOutMax=[]  DifferentiatorOutMin=[]  DifferentiatorOutMax=[]  FilterDiffOutCoefMin=[]  FilterDiffOutCoefMax=[]  ReciprocalOutMin=[]  ReciprocalOutMax=[]  SumDenOutMin=[]  SumDenOutMax=[]  SumNumOutMin=[]  SumNumOutMax=[]  DivideOutMin=[]  DivideOutMax=[]  UdiffTsProdOutMin=[]  UdiffTsProdOutMax=[]  NTsProdOutMin=[]  NTsProdOutMax=[]  UintegralTsProdOutMin=[]  UintegralTsProdOutMax=[]  UngainTsProdOutMin=[]  UngainTsProdOutMax=[]  IntegratorContinuousStateAttributes=''  IntegratorStateMustResolveToSignalObject=off  IntegratorRTWStateStorageClass=Auto  FilterContinuousStateAttributes=''  FilterStateMustResolveToSignalObject=off  FilterRTWStateStorageClass=Auto  ParallelPVariant=InternalParameters  IdealPVariant=Disabled  IVariant=InternalParameters  DVariant=InternalParameters  IntegratorVariant=Continuous  SatVariant=Disabled  AWVariant=Passthrough  PCopyVariant=Disabled  TRVariant=Disabled  FdbkBlocksVariant=Forward  IdealPFdbkVariant=Disabled  SatFdbkVariant=Disabled  DerivativeFilterVariant=ContFilter  NVariant=InternalParameters  NCopyVariant=Disabled  FilterICVariant=InternalICsFilter  IntegratorICVariant=InternalICs  ExternalResetVariant=Disabled  TRSumVariant=Passthrough  SumFdbkVariant=Disabled  SumVariant=Sum_PID  TsampFilterVariant=InternalTs  TsampNgainVariant=Passthrough  TsampIntegralVariant=Passthrough  ExternalSaturationOutDataTypeStr=Inherit: Same as second input
  Sum : Sum  Inputs=|+-
  Sum1 : Sum  Inputs=|+-
  To Workspace : ToWorkspace  VariableName=x_controller  SaveFormat=Timeseries  SampleTime=-1
  To Workspace1 : ToWorkspace  VariableName=y_controller  SaveFormat=Timeseries  SampleTime=-1
  pitch_ref : Outport
  roll_ref : Outport  Port=2
  wires:
  PID Controller1/1 -> Bus Creator1/1, roll_ref/1  "roll_ref"
  yaw/1 -> Error to Body Frame/5(psi)
  Error to Body Frame/1(xbe) -> PID Controller2/1, Bus Creator/3  "xbe"
  u/1 -> Bus Creator/5, Sum/2
  y_ref/1 -> Bus Creator1/6, Error to Body Frame/2(yc)
  Bus Creator/1 -> To Workspace/1
  Sum1/1 -> PID Controller1/1, Bus Creator1/2  "v_ref"
  x/1 -> Bus Creator/2, Error to Body Frame/3(x)
  Bus Creator1/1 -> To Workspace1/1
  PID Controller/1 -> pitch_ref/1, Bus Creator/7  "pitch_ref"
  Sum/1 -> PID Controller/1, Bus Creator/6  "ue"
  x_ref/1 -> Bus Creator/1, Error to Body Frame/1(xc)
  PID Controller2/1 -> Bus Creator/4, Sum/1  "uc"
  y/1 -> Bus Creator1/7, Error to Body Frame/4(y)
  Error to Body Frame/2(ybe) -> PID Controller3/1, Bus Creator1/5  "ybe"
  v/1 -> Sum1/2, Bus Creator1/3
  PID Controller3/1 -> Bus Creator1/4, Sum1/1  "vc"

== system Crazyflie_NoLinealModel_EB/Off-board Controllers [100Hz]/Yaw Controller ==
  yaw_ref : Inport
  yaw : Inport  Port=2
  Enable : EnablePort
  Bus Creator : BusCreator  Inputs=4
  Gain6 : Gain  Gain=180/pi
  PID Controller : pid_lib/PID Controller  Controller=PID  Form=Parallel  TimeDomain=Continuous-time  UseExternalTs=off  SampleTime=-1  IntegratorMethod=Forward Euler  FilterMethod=Forward Euler  ControllerParametersSource=internal  P=Yaw_s(1)  I=Yaw_s(2)  D=Yaw_s(3)  UseFilter=on  N=100  TunerSelectOption=Transfer Function Based (PID Tuner App)  InitialConditionSource=internal  InitialConditionForIntegrator=0  InitialConditionForFilter=0  DifferentiatorICPrevScaledInput=0  ExternalReset=none  TrackingMode=off  Kt=1  LimitOutput=on  SatLimitsSource=internal  UpperSaturationLimit=200  LowerSaturationLimit=-200  LinearizeAsGain=on  AntiWindupMode=none  Kb=1  POutMin=[]  POutMax=[]  IOutMin=[]  IOutMax=[]  DOutMin=[]  DOutMax=[]  NOutMin=[]  NOutMax=[]  SumOutMin=[]  SumOutMax=[]  SaturationOutMin=[]  SaturationOutMax=[]  PParamMin=[]  PParamMax=[]  IParamMin=[]  IParamMax=[]  DParamMin=[]  DParamMax=[]  NParamMin=[]  NParamMax=[]  KbParamMin=[]  KbParamMax=[]  KtParamMin=[]  KtParamMax=[]  KbOutMin=[]  KbOutMax=[]  KtOutMin=[]  KtOutMax=[]  IntegratorOutMin=[]  IntegratorOutMax=[]  FilterOutMin=[]  FilterOutMax=[]  SumI1OutMin=[]  SumI1OutMax=[]  SumI2OutMin=[]  SumI2OutMax=[]  SumI3OutMin=[]  SumI3OutMax=[]  SumI4OutMin=[]  SumI4OutMax=[]  SumDOutMin=[]  SumDOutMax=[]  DifferentiatorOutMin=[]  DifferentiatorOutMax=[]  FilterDiffOutCoefMin=[]  FilterDiffOutCoefMax=[]  ReciprocalOutMin=[]  ReciprocalOutMax=[]  SumDenOutMin=[]  SumDenOutMax=[]  SumNumOutMin=[]  SumNumOutMax=[]  DivideOutMin=[]  DivideOutMax=[]  UdiffTsProdOutMin=[]  UdiffTsProdOutMax=[]  NTsProdOutMin=[]  NTsProdOutMax=[]  UintegralTsProdOutMin=[]  UintegralTsProdOutMax=[]  UngainTsProdOutMin=[]  UngainTsProdOutMax=[]  IntegratorContinuousStateAttributes=''  IntegratorStateMustResolveToSignalObject=off  IntegratorRTWStateStorageClass=Auto  FilterContinuousStateAttributes=''  FilterStateMustResolveToSignalObject=off  FilterRTWStateStorageClass=Auto  ParallelPVariant=InternalParameters  IdealPVariant=Disabled  IVariant=InternalParameters  DVariant=InternalParameters  IntegratorVariant=Continuous  SatVariant=Enabled  AWVariant=Passthrough  PCopyVariant=Disabled  TRVariant=Disabled  FdbkBlocksVariant=Forward  IdealPFdbkVariant=Disabled  SatFdbkVariant=Disabled  DerivativeFilterVariant=ContFilter  NVariant=InternalParameters  NCopyVariant=Disabled  FilterICVariant=InternalICsFilter  IntegratorICVariant=InternalICs  ExternalResetVariant=Disabled  TRSumVariant=Passthrough  SumFdbkVariant=Disabled  SumVariant=Sum_PID  TsampFilterVariant=InternalTs  TsampNgainVariant=Passthrough  TsampIntegralVariant=Passthrough  ExternalSaturationOutDataTypeStr=Inherit: Same as second input
  Sum : Sum  Inputs=|+-
  To Workspace : ToWorkspace  VariableName=yaw_controller  SaveFormat=Timeseries  SampleTime=-1
  dyaw_ref : Outport
  wires:
  PID Controller/1 -> Bus Creator/4, dyaw_ref/1  "control_signal"
  Sum/1 -> PID Controller/1, Bus Creator/3  "yaw_error"
  yaw/1 -> Gain6/1
  yaw_ref/1 -> Bus Creator/1, Sum/1
  Gain6/1 -> Bus Creator/2, Sum/2  "yaw"
  Bus Creator/1 -> To Workspace/1

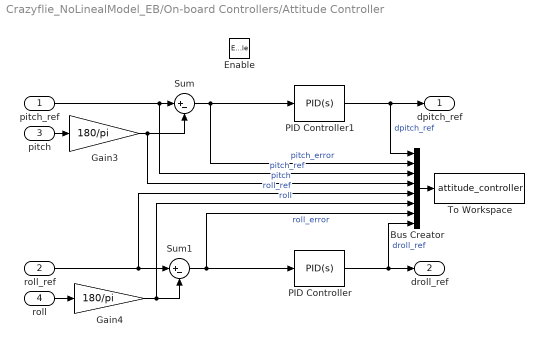
== system Crazyflie_NoLinealModel_EB/On-board Controllers/Attitude Controller ==
  pitch_ref : Inport
  roll_ref : Inport  Port=2
  pitch : Inport  Port=3
  roll : Inport  Port=4
  Enable : EnablePort
  Bus Creator : BusCreator  Inputs=8
  Gain3 : Gain  Gain=180/pi
  Gain4 : Gain  Gain=180/pi
  PID Controller : pid_lib/PID Controller  Controller=PID  Form=Parallel  TimeDomain=Continuous-time  UseExternalTs=off  SampleTime=-1  IntegratorMethod=Forward Euler  FilterMethod=Forward Euler  ControllerParametersSource=internal  P=Theta_s(1)  I=Theta_s(2)  D=Theta_s(3)  UseFilter=on  N=100  TunerSelectOption=Transfer Function Based (PID Tuner App)  InitialConditionSource=internal  InitialConditionForIntegrator=0  InitialConditionForFilter=0  DifferentiatorICPrevScaledInput=0  ExternalReset=none  TrackingMode=off  Kt=1  LimitOutput=on  SatLimitsSource=internal  UpperSaturationLimit=phi_theta_limit  LowerSaturationLimit=-phi_theta_limit  LinearizeAsGain=on  AntiWindupMode=back-calculation  Kb=1/sqrt(Theta_s(2))  POutMin=[]  POutMax=[]  IOutMin=[]  IOutMax=[]  DOutMin=[]  DOutMax=[]  NOutMin=[]  NOutMax=[]  SumOutMin=[]  SumOutMax=[]  SaturationOutMin=[]  SaturationOutMax=[]  PParamMin=[]  PParamMax=[]  IParamMin=[]  IParamMax=[]  DParamMin=[]  DParamMax=[]  NParamMin=[]  NParamMax=[]  KbParamMin=[]  KbParamMax=[]  KtParamMin=[]  KtParamMax=[]  KbOutMin=[]  KbOutMax=[]  KtOutMin=[]  KtOutMax=[]  IntegratorOutMin=[]  IntegratorOutMax=[]  FilterOutMin=[]  FilterOutMax=[]  SumI1OutMin=[]  SumI1OutMax=[]  SumI2OutMin=[]  SumI2OutMax=[]  SumI3OutMin=[]  SumI3OutMax=[]  SumI4OutMin=[]  SumI4OutMax=[]  SumDOutMin=[]  SumDOutMax=[]  DifferentiatorOutMin=[]  DifferentiatorOutMax=[]  FilterDiffOutCoefMin=[]  FilterDiffOutCoefMax=[]  ReciprocalOutMin=[]  ReciprocalOutMax=[]  SumDenOutMin=[]  SumDenOutMax=[]  SumNumOutMin=[]  SumNumOutMax=[]  DivideOutMin=[]  DivideOutMax=[]  UdiffTsProdOutMin=[]  UdiffTsProdOutMax=[]  NTsProdOutMin=[]  NTsProdOutMax=[]  UintegralTsProdOutMin=[]  UintegralTsProdOutMax=[]  UngainTsProdOutMin=[]  UngainTsProdOutMax=[]  IntegratorContinuousStateAttributes=''  IntegratorStateMustResolveToSignalObject=off  IntegratorRTWStateStorageClass=Auto  FilterContinuousStateAttributes=''  FilterStateMustResolveToSignalObject=off  FilterRTWStateStorageClass=Auto  ParallelPVariant=InternalParameters  IdealPVariant=Disabled  IVariant=InternalParameters  DVariant=InternalParameters  IntegratorVariant=Continuous  SatVariant=Enabled  AWVariant=BackCalculation  PCopyVariant=Disabled  TRVariant=Disabled  FdbkBlocksVariant=Forward  IdealPFdbkVariant=Disabled  SatFdbkVariant=Disabled  DerivativeFilterVariant=ContFilter  NVariant=InternalParameters  NCopyVariant=Disabled  FilterICVariant=InternalICsFilter  IntegratorICVariant=InternalICs  ExternalResetVariant=Disabled  TRSumVariant=Passthrough  SumFdbkVariant=Disabled  SumVariant=Sum_PID  TsampFilterVariant=InternalTs  TsampNgainVariant=Passthrough  TsampIntegralVariant=Passthrough  ExternalSaturationOutDataTypeStr=Inherit: Same as second input
  PID Controller1 : pid_lib/PID Controller  Controller=PID  Form=Parallel  TimeDomain=Continuous-time  UseExternalTs=off  SampleTime=-1  IntegratorMethod=Forward Euler  FilterMethod=Forward Euler  ControllerParametersSource=internal  P=Phi_s(1)  I=Phi_s(2)  D=Phi_s(3)  UseFilter=on  N=100  TunerSelectOption=Transfer Function Based (PID Tuner App)  InitialConditionSource=internal  InitialConditionForIntegrator=0  InitialConditionForFilter=0  DifferentiatorICPrevScaledInput=0  ExternalReset=none  TrackingMode=off  Kt=1  LimitOutput=on  SatLimitsSource=internal  UpperSaturationLimit=phi_theta_limit  LowerSaturationLimit=-phi_theta_limit  LinearizeAsGain=on  AntiWindupMode=back-calculation  Kb=1/sqrt(Phi_s(2))  POutMin=[]  POutMax=[]  IOutMin=[]  IOutMax=[]  DOutMin=[]  DOutMax=[]  NOutMin=[]  NOutMax=[]  SumOutMin=[]  SumOutMax=[]  SaturationOutMin=[]  SaturationOutMax=[]  PParamMin=[]  PParamMax=[]  IParamMin=[]  IParamMax=[]  DParamMin=[]  DParamMax=[]  NParamMin=[]  NParamMax=[]  KbParamMin=[]  KbParamMax=[]  KtParamMin=[]  KtParamMax=[]  KbOutMin=[]  KbOutMax=[]  KtOutMin=[]  KtOutMax=[]  IntegratorOutMin=[]  IntegratorOutMax=[]  FilterOutMin=[]  FilterOutMax=[]  SumI1OutMin=[]  SumI1OutMax=[]  SumI2OutMin=[]  SumI2OutMax=[]  SumI3OutMin=[]  SumI3OutMax=[]  SumI4OutMin=[]  SumI4OutMax=[]  SumDOutMin=[]  SumDOutMax=[]  DifferentiatorOutMin=[]  DifferentiatorOutMax=[]  FilterDiffOutCoefMin=[]  FilterDiffOutCoefMax=[]  ReciprocalOutMin=[]  ReciprocalOutMax=[]  SumDenOutMin=[]  SumDenOutMax=[]  SumNumOutMin=[]  SumNumOutMax=[]  DivideOutMin=[]  DivideOutMax=[]  UdiffTsProdOutMin=[]  UdiffTsProdOutMax=[]  NTsProdOutMin=[]  NTsProdOutMax=[]  UintegralTsProdOutMin=[]  UintegralTsProdOutMax=[]  UngainTsProdOutMin=[]  UngainTsProdOutMax=[]  IntegratorContinuousStateAttributes=''  IntegratorStateMustResolveToSignalObject=off  IntegratorRTWStateStorageClass=Auto  FilterContinuousStateAttributes=''  FilterStateMustResolveToSignalObject=off  FilterRTWStateStorageClass=Auto  ParallelPVariant=InternalParameters  IdealPVariant=Disabled  IVariant=InternalParameters  DVariant=InternalParameters  IntegratorVariant=Continuous  SatVariant=Enabled  AWVariant=BackCalculation  PCopyVariant=Disabled  TRVariant=Disabled  FdbkBlocksVariant=Forward  IdealPFdbkVariant=Disabled  SatFdbkVariant=Disabled  DerivativeFilterVariant=ContFilter  NVariant=InternalParameters  NCopyVariant=Disabled  FilterICVariant=InternalICsFilter  IntegratorICVariant=InternalICs  ExternalResetVariant=Disabled  TRSumVariant=Passthrough  SumFdbkVariant=Disabled  SumVariant=Sum_PID  TsampFilterVariant=InternalTs  TsampNgainVariant=Passthrough  TsampIntegralVariant=Passthrough  ExternalSaturationOutDataTypeStr=Inherit: Same as second input
  Sum : Sum  Inputs=|+-
  Sum1 : Sum  Inputs=|+-
  To Workspace : ToWorkspace  VariableName=attitude_controller  SaveFormat=Timeseries  SampleTime=-1
  dpitch_ref : Outport
  droll_ref : Outport  Port=2
  wires:
  pitch_ref/1 -> Bus Creator/3, Sum/1  "pitch_ref"
  Gain4/1 -> Bus Creator/6, Sum1/2  "roll"
  Sum/1 -> PID Controller1/1, Bus Creator/2  "pitch_error"
  roll_ref/1 -> Bus Creator/5, Sum1/1  "roll_ref"
  roll/1 -> Gain4/1
  Gain3/1 -> Bus Creator/4, Sum/2  "pitch"
  pitch/1 -> Gain3/1
  PID Controller1/1 -> Bus Creator/1, dpitch_ref/1  "dpitch_ref"
  Bus Creator/1 -> To Workspace/1
  PID Controller/1 -> Bus Creator/8, droll_ref/1  "droll_ref"
  Sum1/1 -> PID Controller/1, Bus Creator/7  "roll_error"
